simulink model "quad_modell"  (R2015a)
settings: Solver=ode45  StartTime=0.0  StopTime=10.0  RelTol=1e-3
settings Model: Creator=USER  LastModifiedBy=USER

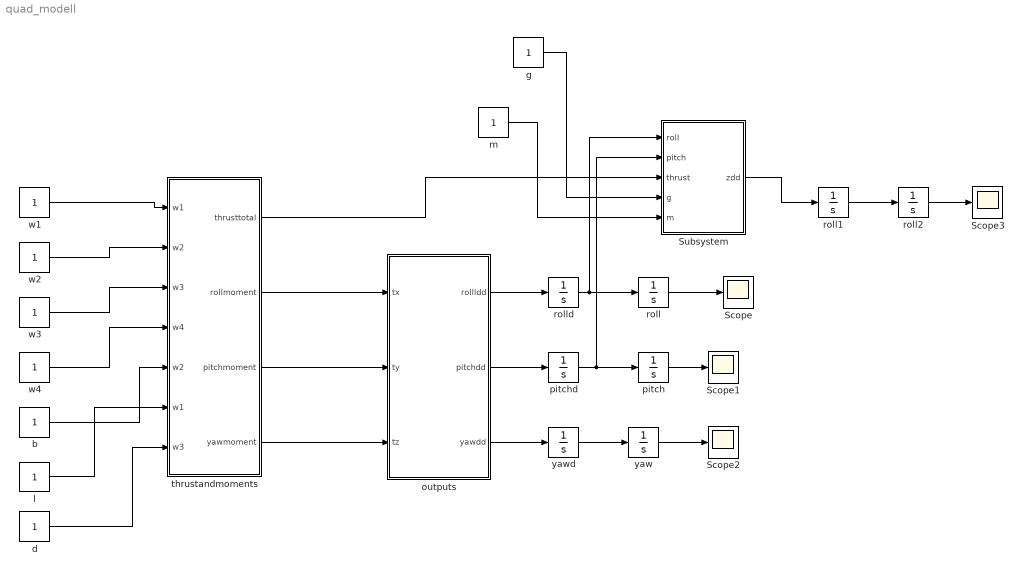
== system quad_modell ==
  Scope{,1..3} (4 alike) : Scope
      Scope2 settings: SaveName=ScopeData2
      Scope3 settings: SaveName=ScopeData3
  Subsystem : Subsystem
  b : Constant
  d : Constant
  g : Constant
  l : Constant
  m : Constant
  outputs : Subsystem
  pitch : Integrator
  pitchd : Integrator
  roll : Integrator
  roll1 : Integrator
  roll2 : Integrator
  rolld : Integrator
  thrustandmoments : Subsystem
  w{1..4} (4 alike) : Constant
  yaw : Integrator
  yawd : Integrator
  wires:
  w1/1 -> thrustandmoments/1("w1 ")
  w2/1 -> thrustandmoments/2("w2 ")
  w3/1 -> thrustandmoments/3("w3 ")
  w4/1 -> thrustandmoments/4(w4)
  b/1 -> thrustandmoments/5(w2)
  l/1 -> thrustandmoments/6(w1)
  d/1 -> thrustandmoments/7(w3)
  outputs/1(rollldd) -> rolld/1
  rolld/1 -> Subsystem/1(roll), roll/1
  outputs/2(pitchdd) -> pitchd/1
  pitchd/1 -> Subsystem/2(pitch), pitch/1
  outputs/3(yawdd) -> yawd/1
  yawd/1 -> yaw/1
  roll/1 -> Scope/1
  pitch/1 -> Scope1/1
  yaw/1 -> Scope2/1
  thrustandmoments/1(thrusttotal) -> Subsystem/3(thrust)
  thrustandmoments/2(rollmoment) -> outputs/1("tx ")
  thrustandmoments/3(pitchmoment) -> outputs/2("ty ")
  thrustandmoments/4(yawmoment) -> outputs/3("tz ")
  Subsystem/1(zdd) -> roll1/1
  roll1/1 -> roll2/1
  roll2/1 -> Scope3/1
  g/1 -> Subsystem/4(g)
  m/1 -> Subsystem/5(m)

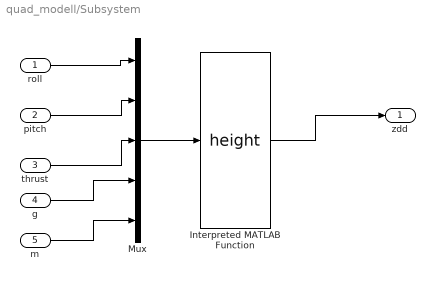
== system quad_modell/Subsystem ==
  roll : Inport
  pitch : Inport  Port=2
  thrust : Inport  Port=3
  g : Inport  Port=4
  m : Inport  Port=5
  "Interpreted MATLAB Function " : MATLABFcn  MATLABFcn=height  OutputDimensions=1  Output1D=off
  Mux : Mux  Inputs=5
  zdd : Outport
  wires:
  roll/1 -> Mux/1
  pitch/1 -> Mux/2
  "Interpreted MATLAB Function "/1 -> zdd/1
  thrust/1 -> Mux/3
  g/1 -> Mux/4
  m/1 -> Mux/5
  Mux/1 -> "Interpreted MATLAB Function "/1

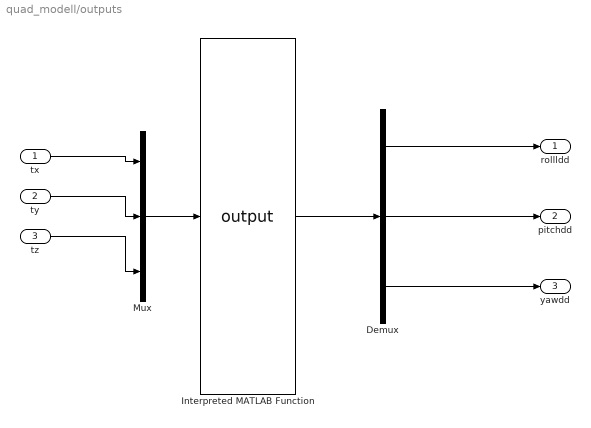
== system quad_modell/outputs ==
  "tx " : Inport
  "ty " : Inport  Port=2
  "tz " : Inport  Port=3
  Demux : Demux  Outputs=3
  Interpreted MATLAB Function : MATLABFcn  MATLABFcn=output  OutputDimensions=3  Output1D=off
  Mux : Mux  Inputs=3
  rollldd : Outport
  pitchdd : Outport  Port=2
  yawdd : Outport  Port=3
  wires:
  "tx "/1 -> Mux/1
  "ty "/1 -> Mux/2
  "tz "/1 -> Mux/3
  Interpreted MATLAB Function/1 -> Demux/1
  Demux/1 -> rollldd/1
  Demux/2 -> pitchdd/1
  Demux/3 -> yawdd/1
  Mux/1 -> Interpreted MATLAB Function/1

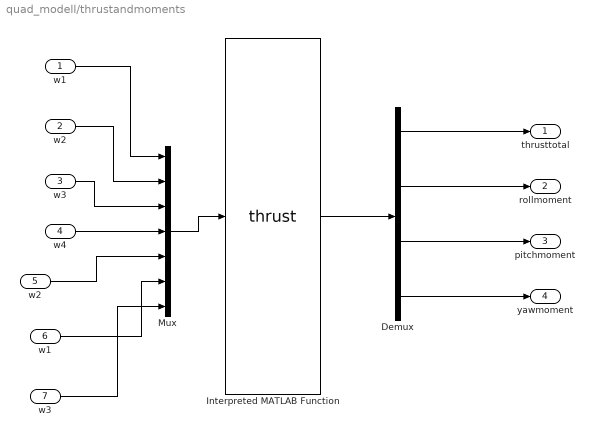
== system quad_modell/thrustandmoments ==
  "w1 " : Inport
  "w2 " : Inport  Port=2
  "w3 " : Inport  Port=3
  w4 : Inport  Port=4
  w2 : Inport  Port=5
  w1 : Inport  Port=6
  w3 : Inport  Port=7
  Demux : Demux
  Interpreted MATLAB Function : MATLABFcn  MATLABFcn=thrust
  Mux : Mux  Inputs=7
  thrusttotal : Outport
  rollmoment : Outport  Port=2
  pitchmoment : Outport  Port=3
  yawmoment : Outport  Port=4
  wires:
  "w1 "/1 -> Mux/1
  "w2 "/1 -> Mux/2
  "w3 "/1 -> Mux/3
  w4/1 -> Mux/4
  Interpreted MATLAB Function/1 -> Demux/1
  Demux/1 -> thrusttotal/1
  Demux/2 -> rollmoment/1
  Demux/3 -> pitchmoment/1
  Mux/1 -> Interpreted MATLAB Function/1
  Demux/4 -> yawmoment/1
  w3/1 -> Mux/7
  w1/1 -> Mux/6
  w2/1 -> Mux/5
